simulink model "Samolot"  (R2022b)
settings: Solver=VariableStepAuto  StartTime=0.0  StopTime=20  RelTol=1e-3
values from neighbouring files (symbols this model uses):
  f_y3_table = [833 400 160 320 520 520 660 830 1070 1600 2100 2800 4100 5000 9000 9000]    [Samolot.m]
  h = 42    [Samolot.m]
  k1 = 54700    [Samolot.m]
  k2 = 303600    [Samolot.m]
  m1 = 14000    [Samolot.m]
  m2 = 450.28    [Samolot.m]
  m3 = 200    [Samolot.m]
  y3_table = [0:10:90, [94 98 102 104 107 120]]    [Samolot.m]
settings Model: Creator=Jakub  LastModifiedBy=Jakub

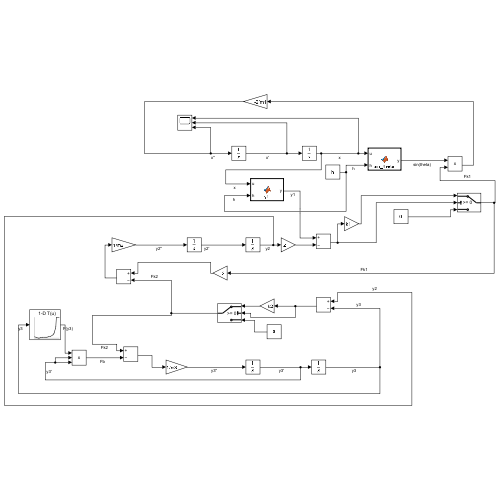
[thumbnail: Simulink's stored preview of the top-level diagram]
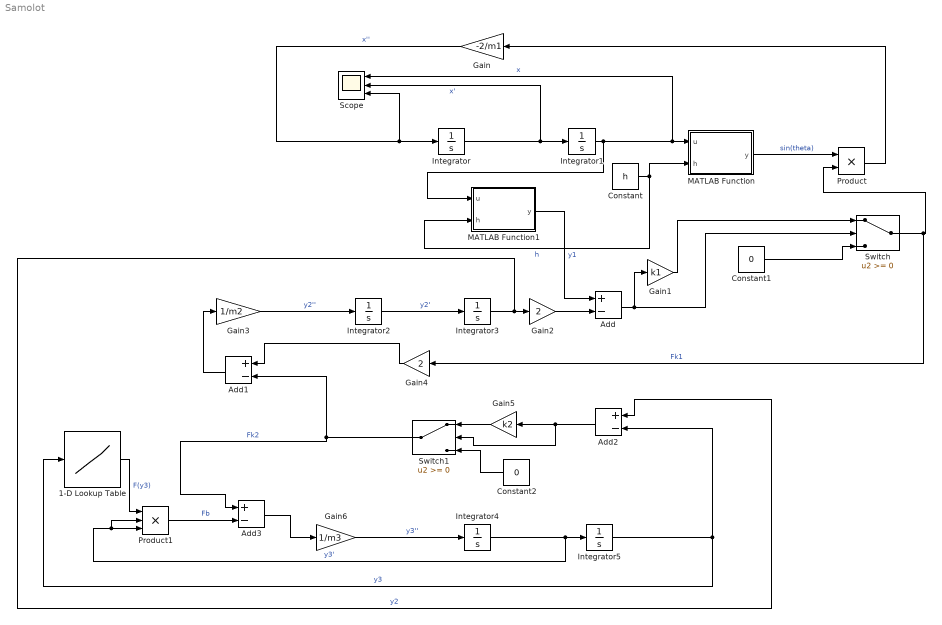
== system Samolot ==
  1-D Lookup Table : Lookup_n-D  NumberOfTableDimensions=1  BreakpointsForDimension1=y3_table  Table=f_y3_table  InternalRulePriority=Speed  RndMeth=Simplest
  Add{,1..3} (4 alike) : Sum  Inputs=+-
  Constant : Constant  Value=h
  Constant1 : Constant  Value=0
  Constant2 : Constant  Value=0
  Gain : Gain  Gain=-2/m1
  Gain1 : Gain  Gain=k1
  Gain2 : Gain  Gain=2
  Gain3 : Gain  Gain=1/m2
  Gain4 : Gain  Gain=2
  Gain5 : Gain  Gain=k2
  Gain6 : Gain  Gain=1/m3
  Integrator : Integrator  InitialCondition=67
  Integrator{1..5} (5 alike) : Integrator
  MATLAB Function : MATLAB Function  TreatAsAtomicUnit=on
  MATLAB Function1 : MATLAB Function  TreatAsAtomicUnit=on
  Product : Product
  Product1 : Product  Inputs=3
  Scope : Scope  NumInputPorts=3
  Switch : Switch  SaturateOnIntegerOverflow=off  InputSameDT=off
  Switch1 : Switch  SaturateOnIntegerOverflow=off  InputSameDT=off
  wires:
  Integrator/1 -> Scope/2, Integrator1/1  "x'"
  Integrator2/1 -> Integrator3/1  "y2'"
  Integrator4/1 -> Product1/2, Product1/3, Integrator5/1  "y3'"
  Gain/1 -> Scope/3, Integrator/1  "x''"
  Integrator1/1 -> Scope/1, MATLAB Function/1(u), MATLAB Function1/1(u)  "x"
  Integrator3/1 -> Gain2/1, Add2/1  "y2"
  Gain3/1 -> Integrator2/1  "y2''"
  Gain6/1 -> Integrator4/1  "y3''"
  Integrator5/1 -> Add2/2, 1-D Lookup Table/1  "y3"
  Constant/1 -> MATLAB Function1/2(h), MATLAB Function/2(h)  "h"
  MATLAB Function/1(y) -> Product/1  "sin(theta)"
  Product/1 -> Gain/1
  Switch/1 -> Gain4/1, Product/2  "Fk1"
  Gain1/1 -> Switch/1
  MATLAB Function1/1(y) -> Add/1  "y1"
  Add/1 -> Gain1/1, Switch/2
  Gain2/1 -> Add/2
  Constant1/1 -> Switch/3
  Add1/1 -> Gain3/1
  Gain4/1 -> Add1/1
  Switch1/1 -> Add1/2, Add3/1  "Fk2"
  Constant2/1 -> Switch1/3
  Add2/1 -> Switch1/2, Gain5/1
  Gain5/1 -> Switch1/1
  Add3/1 -> Gain6/1
  1-D Lookup Table/1 -> Product1/1  "F(y3)"
  Product1/1 -> Add3/2  "Fb"

== matlab function Samolot/MATLAB Function ==
  data: u input; y output; h input
function y = sin_theta(u, h)

    y = u/sqrt(u^2 + h^2);

end

== matlab function Samolot/MATLAB Function1 ==
  data: u input; y output; h input
function y = y1(u, h)

y = sqrt(h^2+u^2) - h;

end
